simulink model "FM_SDR_Receiver_Delay_Line"  (R2019a)
settings: Solver=FixedStepDiscrete  StartTime=0.0  StopTime=inf  RelTol=1e-3
libraries: dspsigops x3, dspsnks4 x1, dsparch4 x1, sdrrlib x1
settings Model: Creator=Kate  LastModifiedBy=Kate

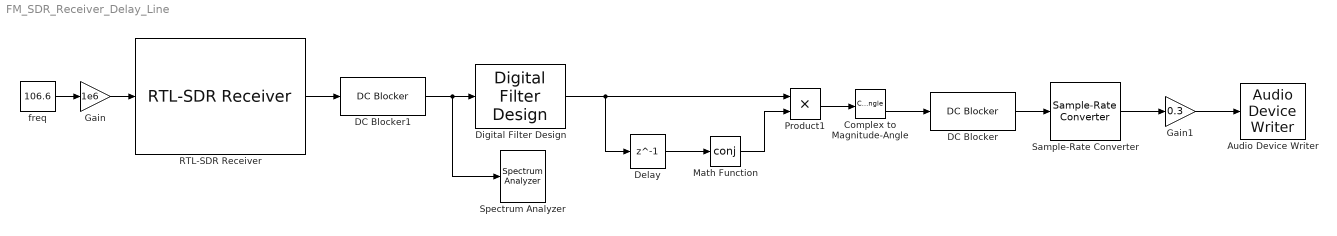
== system FM_SDR_Receiver_Delay_Line ==
  Audio Device Writer : dspsnks4/Audio Device Writer  Driver=DirectSound  Device=Default  InheritSampleRate=on  SampleRate=44100  BitDepth=16-bit integer  BufferSize=4096  NumBuffers=10  DefaultOutputChannelMapping=on  OutputChannelMapping=1:2  OutputNumUnderrunSamples=off  DriverIdx=1  DeviceWarnFlag=''
  Complex to Magnitude-Angle : ComplexToMagnitudeAngle
  DC Blocker : dspsigops/DC Blocker  Algorithm=IIR  NormalizedBandwidth=0.001  Length=50  Order=6  SimulateUsing=Code generation
      settings: SourceProductName=DSP System Toolbox  SourceProductBaseCode=DS
  DC Blocker1 : dspsigops/DC Blocker  Algorithm=IIR  NormalizedBandwidth=0.001  Length=50  Order=6  SimulateUsing=Code generation
      settings: SourceProductName=DSP System Toolbox  SourceProductBaseCode=DS
  Delay : Delay  DelayLength=1  InputProcessing=Columns as channels (frame based)
  Digital Filter Design : dsparch4/Digital Filter Design  mwdsp_browser_bugfix_var=off
  Gain : Gain  Gain=1e6
  Gain1 : Gain  Gain=0.3
  Math Function : Math  Operator=conj  SaturateOnIntegerOverflow=on
  Product1 : Product
  RTL-SDR Receiver : sdrrlib/RTL-SDR Receiver  IPAddress=0  CenterFrequencySource=Input port  CenterFrequency=102.5e6  GainSource=AGC  Gain=0  ADCRate=1.2e6  FrequencyCorrection=0  LostSamplesOutputPort=off  LatencyOutputPort=off  OutputDataType=double  FrameLength=512*25  EnableBurstMode=off  NumFramesInBurst=20  sobjType=sdrr.internal.SDRRTLReceiverSL  dataUDPPort=-1  ctrlUDPPort=-1  subDeviceList=nosubdev  sdrBlockType=SDRBlockTypeSLT.SDRRxBlock  requester=UNUSED_BY_SFCN  sdrExecutionMode=SDRExecutionModeSLT.ExecModeHW  BypassUserLogic=off  DecimatorSelect=DDC decimator  SourceSelect=RF data  SineAmplitude=16000  EnableInternalClock=off  BypassIQBalance=off  IFBandwidth=40e6  ADCRateSource=Dialog  IntermediateFrequency=0  DecimationFactorSource=Dialog  DecimationFactor=512  RFFrequencyIsTunable=logical(1)  SampleTime=(512*25)/(1.2e6)  IFBandwidthSource=Dialog  SineFrequency=30000  BypassDCBlockingFilter=off  IntermediateFrequencySource=Dialog  IQBalanceCoefficients=64  SkipAllHardwareResetAndInitialization=off  EnableIQCalibrationTable=on  CacheIQCalibrationTable=off  EnableOffsetTuning=off  EnableRTLAGC=off  EnableTestMode=off  EnableTunerAGC=on  FrequencyCorrectionSource=Dialog  NumMLBuffers=128  NumUSBBuffers=16  RTLCrystalFrequency=28800000  TunerCrystalFrequency=28800000
      settings: SourceProductName=Communications Toolbox Support Package for RTL-SDR Radio  SourceProductBaseCode=RTLSDR
  Sample-Rate Converter : dspsigops/Sample-Rate Converter  InputSampleRate=1.2e6  OutputSampleRate=48e3  OutputRateTolerance=0  Bandwidth=30e3  StopbandAttenuation=80  SimulateUsing=Code generation
      settings: SourceProductName=DSP System Toolbox  SourceProductBaseCode=DS
  Spectrum Analyzer : SpectrumAnalyzer
  freq : Constant  Value=106.6
  wires:
  freq/1 -> Gain/1
  Gain/1 -> RTL-SDR Receiver/1
  Product1/1 -> Complex to Magnitude-Angle/1
  Gain1/1 -> Audio Device Writer/1
  RTL-SDR Receiver/1 -> DC Blocker1/1
  DC Blocker1/1 -> Spectrum Analyzer/1, Digital Filter Design/1
  Delay/1 -> Math Function/1
  Sample-Rate Converter/1 -> Gain1/1
  DC Blocker/1 -> Sample-Rate Converter/1
  Math Function/1 -> Product1/2
  Complex to Magnitude-Angle/2 -> DC Blocker/1
  Digital Filter Design/1 -> Product1/1, Delay/1
